simulink model "ProvaEffetti"  (R2020a)
settings: Solver=VariableStepAuto  StartTime=0.0  StopTime=Inf  RelTol=1e-3
libraries: audiodynamicrange x2, audiosources x1, dspsnks4 x1, audioeffects x1
settings Model: Creator=miche  LastModifiedBy=miche

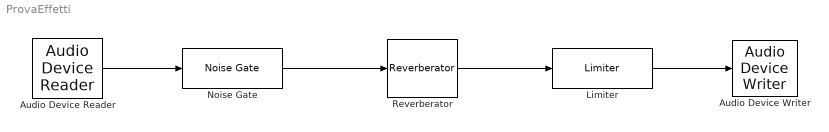
== system ProvaEffetti ==
  Audio Device Reader : audiosources/Audio Device Reader  Driver=DirectSound  Device=Default  SampleRate=44100  NumChannels=1  SamplesPerFrame=1024  BitDepth=16-bit integer  NumBuffers=10  DefaultInputChannelMapping=on  InputChannelMapping=1:2  OutputNumOverrunSamples=off  OutputDataType=double  DriverIdx=1  DeviceWarnFlag=''
      settings: SourceProductBaseCode=AU
  Audio Device Writer : dspsnks4/Audio Device Writer  Driver=DirectSound  Device=Default  InheritSampleRate=on  SampleRate=44100  BitDepth=16-bit integer  BufferSize=4096  NumBuffers=10  DefaultOutputChannelMapping=on  OutputChannelMapping=1:2  OutputNumUnderrunSamples=off  DriverIdx=1  DeviceWarnFlag=''
  Limiter : audiodynamicrange/Limiter  ThresholdPort=off  Threshold=0.0  KneeWidthPort=off  KneeWidth=0.0  AttackTimePort=off  AttackTime=0.0  ReleaseTimePort=off  ReleaseTime=0.2  MakeUpGainMode=Property  MakeUpGain=0.0  InheritSampleRate=on  SampleRate=44100  outputGain=off  SimulateUsing=Code generation
      settings: SourceProductBaseCode=AU
  Noise Gate : audiodynamicrange/Noise Gate  ThresholdPort=off  Threshold=-100  AttackTimePort=off  AttackTime=0.05  ReleaseTimePort=off  ReleaseTime=0.2  HoldTimePort=off  HoldTime=0.05  InheritSampleRate=on  SampleRate=44100  outputGain=off  SimulateUsing=Code generation
      settings: SourceProductBaseCode=AU
  Reverberator : audioeffects/Reverberator  PreDelayPort=off  PreDelay=0  HighCutFrequencyPort=off  HighCutFrequency=20000  DiffusionPort=off  Diffusion=0.75  DecayFactorPort=off  DecayFactor=0.60  HighFrequencyDampingPort=off  HighFrequencyDamping=0.0005  WetDryMixPort=off  WetDryMix=0.500  InheritSampleRate=on  SampleRate=44100  SimulateUsing=Interpreted execution
      settings: SourceProductBaseCode=AU
  wires:
  Noise Gate/1 -> Reverberator/1
  Reverberator/1 -> Limiter/1
  Audio Device Reader/1 -> Noise Gate/1
  Limiter/1 -> Audio Device Writer/1
